simulink model "blockdemo_preaddermodes"  (Simulink 7.6)
settings: Solver=ode45  StartTime=0.0  StopTime=10.0  RelTol=1e-3
InitFcn:
  | %% DSPBuilder Start
  | alt_dspbuilder_update_model(bdroot)
  | %% DSPBuilder End
libraries: allblocks_alteradspbuilder2 x19
settings Model: Creator=akarapet  LastModifiedBy=akarapet

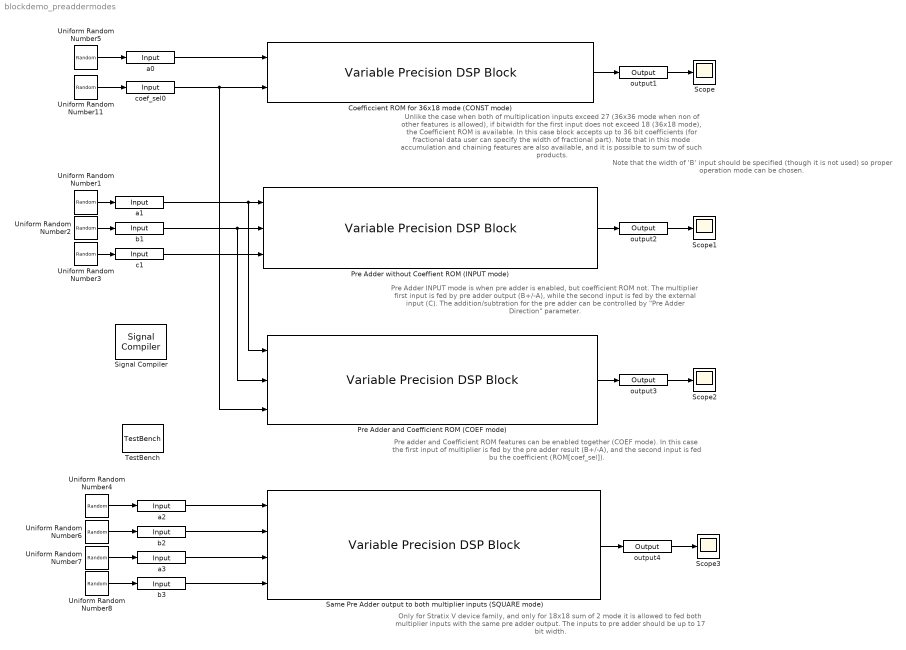
== system blockdemo_preaddermodes ==
  note: Unlike the case when both of multiplication inputs exceed 27 (36x36 mode when non of other features is allowed),
      | if bitwidth for the first input does not exceed 18 (36x18 mode), the Coefficient ROM is available.
      | In this case block accepts up to 36 bit coefficients (for fractional data user can specify the width of fractional part).
      | Note that in this mode accumulation and chaining features are also available, and it is possible to sum tw of such products.
  note: Note that the width of 'B' input should be specified (though it is not used) so proper operation mode can be chosen.
  note: Pre Adder INPUT mode is when pre adder is enabled, but coefficient ROM not. The multiplier first input is fed by
      | pre adder output (B+/-A), while the second input is fed by the external input (C).
      | The addition/subtration for the pre adder can be controlled by "Pre Adder Direction" parameter.
  note: Pre adder and Coefficient ROM features can be enabled together (COEF mode). In this case the first input
      | of multiplier is fed by the pre adder result (B+/-A), and the second input is fed bu the coefficient (ROM[coef_sel]).
  note: Only for Stratix V device family, and only for 18x18 sum of 2 mode it is allowed to fed
      | both multiplier inputs with the same pre adder output.
      | The inputs to pre adder should be up to 17 bit width.
  Coefficcient ROM for 36x18 mode (CONST mode) : allblocks_alteradspbuilder2/Variable Precision DSP Block  complex_model_delayed=0  model_delayed=0  device_family=Stratix V  used_mode_stratix=Other Modes  used_mode_arria=Other Modes  in_25x18_complex_mode=0  in_18x18plus36_mode=0  in_other_modes=1  number_of_mults=1  clock_ena_inputs=off  async_clear_inputs=off  bus_type=Signed Integer  bwl_A=18  bwr_A=0  width_A=18  chain_width=64  reg_inputs_A=off  A_inputs_reg_ena=ENABLE 0  bwl_B=36  bwr_B=0  width_B=36  reg_inputs_B=off  B_inputs_reg_ena=ENABLE 0  bwl_joint_A_B=8  bwr_joint_A_B=0  reg_joint_A_B_input=on  A_B_input_reg_ena=ENABLE 0  bwl_A_complex=8  bwr_A_complex=8  reg_complex_A=on  A_complex_inputs_reg_ena=ENABLE 0  bwl_B_complex=8  bwr_B_complex=8  reg_complex_B=on  B_complex_inputs_reg_ena=ENABLE 0  A_inputs_exist=1  B_inputs_exist=0  C_inputs_exist=0  coef_sel_inputs_exist=1  all_inputs_registered=0  no_input_registered=1  all_inputs_share_same_clocks=1  full_resolution=off  bwl_out=54  bwr_out=0  reg_output=off  output_reg_ena=ENABLE 0  systolic_regs_available=0  enable_systolic_regs=off  systolic_regs_used=0  basic_struct_ok_for_input_scan=0  input_scan_available=0  enable_input_scan=off  input_scan_used=0  input_scan_delay_regs_available=0  enable_input_scan_delay_regs=off  input_scan_delay_regs_used=0  basic_struct_ok_for_coef_rom=1  coef_rom_available=1  enable_coef_rom=on  coef_rom_used=1  basic_struct_ok_for_preadder=0  preadder_available=0  enable_preadder=off  preadder_used=0  preadder_direction=ADD  square_mode_available=0  enable_square_mode=off  square_mode_used=0  upper_limit_9bit=9  upper_limit_18bit=18  upper_limit_27bit=27  in_18x18_modes=0  in_27x27_modes=0  in_36x18_modes=1  in_36x36_mode=0  mult1_adder_available=0  mult1_direction=ADD  mult3_adder_available=0  mult3_direction=ADD  chainout_adder_available=1  use_chainout_input=off  chainout_input_used=0  use_chainout_output=off  chainout_output_used=0  accum_available=1  enable_accum=off  accum_used=0  double_accum_available=0  enable_double_accum=off  double_accum_used=0  negate_available=1  mult_add_operation=ADD  rounding_constant_available=1  use_rounding_constant=off  rounding_constant_used=0  constant_value=1  bwl_C=8  bwr_C=0  bwl_coef=36  bwr_coef=0  mult0_coeffs=[2147483648, -2147483648, -211, 0, 7, 44, -2147483630, 333]  mult1_coeffs=[0, 0, 0, 0, 0, 0, 0, 0]  mult2_coeffs=[0, 0, 0, 0, 0, 0, 0, 0]  mult3_coeffs=[0, 0, 0, 0, 0, 0, 0, 0]  reg_mult1_op_control=off  reg_mult3_op_control=off  reg_accum_control=off  reg_negate_control=off  control_regs_ena=ENABLE 0
  Pre Adder and Coefficient ROM (COEF mode) : allblocks_alteradspbuilder2/Variable Precision DSP Block  complex_model_delayed=0  model_delayed=0  device_family=Stratix V  used_mode_stratix=Other Modes  used_mode_arria=Other Modes  in_25x18_complex_mode=0  in_18x18plus36_mode=0  in_other_modes=1  number_of_mults=1  clock_ena_inputs=off  async_clear_inputs=off  bus_type=Signed Integer  bwl_A=20  bwr_A=0  width_A=20  chain_width=64  reg_inputs_A=on  A_inputs_reg_ena=ENABLE 0  bwl_B=20  bwr_B=0  width_B=20  reg_inputs_B=on  B_inputs_reg_ena=ENABLE 0  bwl_joint_A_B=8  bwr_joint_A_B=0  reg_joint_A_B_input=on  A_B_input_reg_ena=ENABLE 0  bwl_A_complex=8  bwr_A_complex=8  reg_complex_A=on  A_complex_inputs_reg_ena=ENABLE 0  bwl_B_complex=8  bwr_B_complex=8  reg_complex_B=on  B_complex_inputs_reg_ena=ENABLE 0  A_inputs_exist=1  B_inputs_exist=1  C_inputs_exist=0  coef_sel_inputs_exist=1  all_inputs_registered=1  no_input_registered=0  all_inputs_share_same_clocks=1  full_resolution=off  bwl_out=41  bwr_out=0  reg_output=off  output_reg_ena=ENABLE 0  systolic_regs_available=0  enable_systolic_regs=off  systolic_regs_used=0  basic_struct_ok_for_input_scan=1  input_scan_available=0  enable_input_scan=off  input_scan_used=0  input_scan_delay_regs_available=0  enable_input_scan_delay_regs=off  input_scan_delay_regs_used=0  basic_struct_ok_for_coef_rom=1  coef_rom_available=1  enable_coef_rom=on  coef_rom_used=1  basic_struct_ok_for_preadder=1  preadder_available=1  enable_preadder=on  preadder_used=1  preadder_direction=ADD  square_mode_available=0  enable_square_mode=off  square_mode_used=0  upper_limit_9bit=9  upper_limit_18bit=17  upper_limit_27bit=27  in_18x18_modes=0  in_27x27_modes=1  in_36x18_modes=0  in_36x36_mode=0  mult1_adder_available=0  mult1_direction=ADD  mult3_adder_available=0  mult3_direction=ADD  chainout_adder_available=1  use_chainout_input=off  chainout_input_used=0  use_chainout_output=off  chainout_output_used=0  accum_available=1  enable_accum=off  accum_used=0  double_accum_available=0  enable_double_accum=off  double_accum_used=0  negate_available=1  mult_add_operation=ADD  rounding_constant_available=1  use_rounding_constant=off  rounding_constant_used=0  constant_value=1  bwl_C=20  bwr_C=0  bwl_coef=27  bwr_coef=0  mult0_coeffs=[200, -38, 21, -76, 7, 44, -1, 0]  mult1_coeffs=[0, 0, 0, 0, 0, 0, 0, 0]  mult2_coeffs=[0, 0, 0, 0, 0, 0, 0, 0]  mult3_coeffs=[0, 0, 0, 0, 0, 0, 0, 0]  reg_mult1_op_control=off  reg_mult3_op_control=off  reg_accum_control=off  reg_negate_control=off  control_regs_ena=ENABLE 0
  Pre Adder without Coeffient ROM (INPUT mode) : allblocks_alteradspbuilder2/Variable Precision DSP Block  complex_model_delayed=0  model_delayed=0  device_family=Stratix V  used_mode_stratix=Other Modes  used_mode_arria=Other Modes  in_25x18_complex_mode=0  in_18x18plus36_mode=0  in_other_modes=1  number_of_mults=1  clock_ena_inputs=off  async_clear_inputs=off  bus_type=Signed Integer  bwl_A=20  bwr_A=0  width_A=20  chain_width=64  reg_inputs_A=on  A_inputs_reg_ena=ENABLE 0  bwl_B=20  bwr_B=0  width_B=20  reg_inputs_B=on  B_inputs_reg_ena=ENABLE 0  bwl_joint_A_B=8  bwr_joint_A_B=0  reg_joint_A_B_input=on  A_B_input_reg_ena=ENABLE 0  bwl_A_complex=8  bwr_A_complex=8  reg_complex_A=on  A_complex_inputs_reg_ena=ENABLE 0  bwl_B_complex=8  bwr_B_complex=8  reg_complex_B=on  B_complex_inputs_reg_ena=ENABLE 0  A_inputs_exist=1  B_inputs_exist=1  C_inputs_exist=1  coef_sel_inputs_exist=0  all_inputs_registered=1  no_input_registered=0  all_inputs_share_same_clocks=1  full_resolution=off  bwl_out=41  bwr_out=0  reg_output=on  output_reg_ena=ENABLE 0  systolic_regs_available=0  enable_systolic_regs=off  systolic_regs_used=0  basic_struct_ok_for_input_scan=1  input_scan_available=0  enable_input_scan=off  input_scan_used=0  input_scan_delay_regs_available=0  enable_input_scan_delay_regs=off  input_scan_delay_regs_used=0  basic_struct_ok_for_coef_rom=1  coef_rom_available=1  enable_coef_rom=off  coef_rom_used=0  basic_struct_ok_for_preadder=1  preadder_available=1  enable_preadder=on  preadder_used=1  preadder_direction=ADD  square_mode_available=0  enable_square_mode=off  square_mode_used=0  upper_limit_9bit=9  upper_limit_18bit=17  upper_limit_27bit=27  in_18x18_modes=0  in_27x27_modes=1  in_36x18_modes=0  in_36x36_mode=0  mult1_adder_available=0  mult1_direction=ADD  mult3_adder_available=0  mult3_direction=ADD  chainout_adder_available=1  use_chainout_input=off  chainout_input_used=0  use_chainout_output=off  chainout_output_used=0  accum_available=1  enable_accum=off  accum_used=0  double_accum_available=0  enable_double_accum=off  double_accum_used=0  negate_available=1  mult_add_operation=ADD  rounding_constant_available=1  use_rounding_constant=off  rounding_constant_used=0  constant_value=1  bwl_C=20  bwr_C=0  bwl_coef=27  bwr_coef=0  mult0_coeffs=[0, 0, 0, 0, 0, 0, 0, 0]  mult1_coeffs=[0, 0, 0, 0, 0, 0, 0, 0]  mult2_coeffs=[0, 0, 0, 0, 0, 0, 0, 0]  mult3_coeffs=[0, 0, 0, 0, 0, 0, 0, 0]  reg_mult1_op_control=off  reg_mult3_op_control=off  reg_accum_control=off  reg_negate_control=off  control_regs_ena=ENABLE 0
  Same Pre Adder output to both multiplier inputs (SQUARE mode) : allblocks_alteradspbuilder2/Variable Precision DSP Block  complex_model_delayed=0  model_delayed=0  device_family=Stratix V  used_mode_stratix=Other Modes  used_mode_arria=Other Modes  in_25x18_complex_mode=0  in_18x18plus36_mode=0  in_other_modes=1  number_of_mults=2  clock_ena_inputs=off  async_clear_inputs=off  bus_type=Signed Integer  bwl_A=17  bwr_A=0  width_A=17  chain_width=64  reg_inputs_A=off  A_inputs_reg_ena=ENABLE 0  bwl_B=17  bwr_B=0  width_B=17  reg_inputs_B=off  B_inputs_reg_ena=ENABLE 0  bwl_joint_A_B=8  bwr_joint_A_B=0  reg_joint_A_B_input=on  A_B_input_reg_ena=ENABLE 0  bwl_A_complex=8  bwr_A_complex=8  reg_complex_A=on  A_complex_inputs_reg_ena=ENABLE 0  bwl_B_complex=8  bwr_B_complex=8  reg_complex_B=on  B_complex_inputs_reg_ena=ENABLE 0  A_inputs_exist=1  B_inputs_exist=1  C_inputs_exist=0  coef_sel_inputs_exist=0  all_inputs_registered=0  no_input_registered=1  all_inputs_share_same_clocks=1  full_resolution=off  bwl_out=35  bwr_out=0  reg_output=on  output_reg_ena=ENABLE 0  systolic_regs_available=1  enable_systolic_regs=off  systolic_regs_used=0  basic_struct_ok_for_input_scan=1  input_scan_available=0  enable_input_scan=off  input_scan_used=0  input_scan_delay_regs_available=0  enable_input_scan_delay_regs=off  input_scan_delay_regs_used=0  basic_struct_ok_for_coef_rom=1  coef_rom_available=1  enable_coef_rom=off  coef_rom_used=0  basic_struct_ok_for_preadder=1  preadder_available=1  enable_preadder=on  preadder_used=1  preadder_direction=SUB  square_mode_available=1  enable_square_mode=on  square_mode_used=1  upper_limit_9bit=9  upper_limit_18bit=17  upper_limit_27bit=27  in_18x18_modes=1  in_27x27_modes=0  in_36x18_modes=0  in_36x36_mode=0  mult1_adder_available=1  mult1_direction=ADD  mult3_adder_available=0  mult3_direction=ADD  chainout_adder_available=1  use_chainout_input=off  chainout_input_used=0  use_chainout_output=off  chainout_output_used=0  accum_available=1  enable_accum=off  accum_used=0  double_accum_available=0  enable_double_accum=off  double_accum_used=0  negate_available=1  mult_add_operation=ADD  rounding_constant_available=1  use_rounding_constant=off  rounding_constant_used=0  constant_value=1  bwl_C=20  bwr_C=0  bwl_coef=18  bwr_coef=0  mult0_coeffs=[200, -38, 21, -76, 7, 44, -1, 0]  mult1_coeffs=[0, 0, 0, 0, 0, 0, 0, 0]  mult2_coeffs=[0, 0, 0, 0, 0, 0, 0, 0]  mult3_coeffs=[0, 0, 0, 0, 0, 0, 0, 0]  reg_mult1_op_control=off  reg_mult3_op_control=off  reg_accum_control=off  reg_negate_control=off  control_regs_ena=ENABLE 0
  Scope{,1..3} (4 alike) : Scope
      Scope2 settings: SaveName=ScopeData2
      Scope3 settings: SaveName=ScopeData3
  Signal Compiler : allblocks_alteradspbuilder2/Signal Compiler  DeviceFamily=Stratix V  DeviceName=AUTO  EnableSignalTap=off  SignalTapDepth=128  UseBoardBlock=off  StpUseDefaultClock=on  StpClock=Clock  ExportDir=<binary blob, 153 chars, not shown>
  TestBench : allblocks_alteradspbuilder2/TestBench  enable=on  advancedMode=off  modelSimGui=off  maxDisplayErrors=10  mismatchErrorLevel=Error  simdatafile=/data/akarapet/qshell_linux64_regtests/p4/dsp_builder/dsp_builder2/Documentation/DesignExamples/Tutorials/UnitBlocks/Arithmetic/VariablePrecisionDSPBlock/tb_blockdemo_preaddermodes/blockdemo_preaddermodes.simdata.tcl
  Uniform Random Number{1,4..8} (6 alike) : UniformRandomNumber  Minimum=-2147483642  Maximum=2147483642  Seed=1591  SampleTime=1
  Uniform Random Number11 : UniformRandomNumber  Minimum=0  Maximum=7  Seed=1591  SampleTime=1
  Uniform Random Number2 : UniformRandomNumber  Minimum=-2147483642  Maximum=2147483642  Seed=3333  SampleTime=1
  Uniform Random Number3 : UniformRandomNumber  Minimum=-2147483642  Maximum=2147483642  Seed=3323  SampleTime=1
  a0 : allblocks_alteradspbuilder2/Input  iofile=/data/akarapet/qshell_linux64_regtests/p4/dsp_builder/dsp_builder2/Documentation/DesignExamples/Tutorials/UnitBlocks/Arithmetic/VariablePrecisionDSPBlock/tb_blockdemo_preaddermodes/blockdemo%5Fpreaddermodes_a0.salt  BusType=Signed Integer  bwl=18  bwr=0  SpecifyClock=off  clock=default_clock  PORTTYPE=Input  externalType=Inferred  allowFloatingPointOverride=on  logOutputs=off
  a1 : allblocks_alteradspbuilder2/Input  iofile=/data/akarapet/qshell_linux64_regtests/p4/dsp_builder/dsp_builder2/Documentation/DesignExamples/Tutorials/UnitBlocks/Arithmetic/VariablePrecisionDSPBlock/tb_blockdemo_preaddermodes/blockdemo%5Fpreaddermodes_a1.salt  BusType=Signed Integer  bwl=20  bwr=0  SpecifyClock=off  clock=default_clock  PORTTYPE=Input  externalType=Inferred  allowFloatingPointOverride=on  logOutputs=off
  a2 : allblocks_alteradspbuilder2/Input  iofile=/data/akarapet/qshell_linux64_regtests/p4/dsp_builder/dsp_builder2/Documentation/DesignExamples/Tutorials/UnitBlocks/Arithmetic/VariablePrecisionDSPBlock/tb_blockdemo_preaddermodes/blockdemo%5Fpreaddermodes_a2.salt  BusType=Signed Integer  bwl=17  bwr=0  SpecifyClock=off  clock=default_clock  PORTTYPE=Input  externalType=Inferred  allowFloatingPointOverride=on  logOutputs=off
  a3 : allblocks_alteradspbuilder2/Input  iofile=/data/akarapet/qshell_linux64_regtests/p4/dsp_builder/dsp_builder2/Documentation/DesignExamples/Tutorials/UnitBlocks/Arithmetic/VariablePrecisionDSPBlock/tb_blockdemo_preaddermodes/blockdemo%5Fpreaddermodes_a3.salt  BusType=Signed Integer  bwl=17  bwr=0  SpecifyClock=off  clock=default_clock  PORTTYPE=Input  externalType=Inferred  allowFloatingPointOverride=on  logOutputs=off
  b1 : allblocks_alteradspbuilder2/Input  iofile=/data/akarapet/qshell_linux64_regtests/p4/dsp_builder/dsp_builder2/Documentation/DesignExamples/Tutorials/UnitBlocks/Arithmetic/VariablePrecisionDSPBlock/tb_blockdemo_preaddermodes/blockdemo%5Fpreaddermodes_b1.salt  BusType=Signed Integer  bwl=20  bwr=0  SpecifyClock=off  clock=default_clock  PORTTYPE=Input  externalType=Inferred  allowFloatingPointOverride=on  logOutputs=off
  b2 : allblocks_alteradspbuilder2/Input  iofile=/data/akarapet/qshell_linux64_regtests/p4/dsp_builder/dsp_builder2/Documentation/DesignExamples/Tutorials/UnitBlocks/Arithmetic/VariablePrecisionDSPBlock/tb_blockdemo_preaddermodes/blockdemo%5Fpreaddermodes_b2.salt  BusType=Signed Integer  bwl=17  bwr=0  SpecifyClock=off  clock=default_clock  PORTTYPE=Input  externalType=Inferred  allowFloatingPointOverride=on  logOutputs=off
  b3 : allblocks_alteradspbuilder2/Input  iofile=/data/akarapet/qshell_linux64_regtests/p4/dsp_builder/dsp_builder2/Documentation/DesignExamples/Tutorials/UnitBlocks/Arithmetic/VariablePrecisionDSPBlock/tb_blockdemo_preaddermodes/blockdemo%5Fpreaddermodes_b3.salt  BusType=Signed Integer  bwl=17  bwr=0  SpecifyClock=off  clock=default_clock  PORTTYPE=Input  externalType=Inferred  allowFloatingPointOverride=on  logOutputs=off
  c1 : allblocks_alteradspbuilder2/Input  iofile=/data/akarapet/qshell_linux64_regtests/p4/dsp_builder/dsp_builder2/Documentation/DesignExamples/Tutorials/UnitBlocks/Arithmetic/VariablePrecisionDSPBlock/tb_blockdemo_preaddermodes/blockdemo%5Fpreaddermodes_c1.salt  BusType=Signed Integer  bwl=20  bwr=0  SpecifyClock=off  clock=default_clock  PORTTYPE=Input  externalType=Inferred  allowFloatingPointOverride=on  logOutputs=off
  coef_sel0 : allblocks_alteradspbuilder2/Input  iofile=/data/akarapet/qshell_linux64_regtests/p4/dsp_builder/dsp_builder2/Documentation/DesignExamples/Tutorials/UnitBlocks/Arithmetic/VariablePrecisionDSPBlock/tb_blockdemo_preaddermodes/blockdemo%5Fpreaddermodes_coef%5Fsel0.salt  BusType=Unsigned Integer  bwl=3  bwr=0  SpecifyClock=off  clock=default_clock  PORTTYPE=Input  externalType=Inferred  allowFloatingPointOverride=on  logOutputs=off
  output1 : allblocks_alteradspbuilder2/Output  iofile=/data/akarapet/qshell_linux64_regtests/p4/dsp_builder/dsp_builder2/Documentation/DesignExamples/Tutorials/UnitBlocks/Arithmetic/VariablePrecisionDSPBlock/tb_blockdemo_preaddermodes/blockdemo%5Fpreaddermodes_output1.capture  BusType=Signed Integer  bwl=54  bwr=0  externalType=Inferred  PORTTYPE=Output  allowFloatingPointOverride=on  logOutputs=off
  output2 : allblocks_alteradspbuilder2/Output  iofile=/data/akarapet/qshell_linux64_regtests/p4/dsp_builder/dsp_builder2/Documentation/DesignExamples/Tutorials/UnitBlocks/Arithmetic/VariablePrecisionDSPBlock/tb_blockdemo_preaddermodes/blockdemo%5Fpreaddermodes_output2.capture  BusType=Signed Integer  bwl=41  bwr=0  externalType=Inferred  PORTTYPE=Output  allowFloatingPointOverride=on  logOutputs=off
  output3 : allblocks_alteradspbuilder2/Output  iofile=/data/akarapet/qshell_linux64_regtests/p4/dsp_builder/dsp_builder2/Documentation/DesignExamples/Tutorials/UnitBlocks/Arithmetic/VariablePrecisionDSPBlock/tb_blockdemo_preaddermodes/blockdemo%5Fpreaddermodes_output3.capture  BusType=Signed Integer  bwl=41  bwr=0  externalType=Inferred  PORTTYPE=Output  allowFloatingPointOverride=on  logOutputs=off
  output4 : allblocks_alteradspbuilder2/Output  iofile=/data/akarapet/qshell_linux64_regtests/p4/dsp_builder/dsp_builder2/Documentation/DesignExamples/Tutorials/UnitBlocks/Arithmetic/VariablePrecisionDSPBlock/tb_blockdemo_preaddermodes/blockdemo%5Fpreaddermodes_output4.capture  BusType=Signed Integer  bwl=35  bwr=0  externalType=Inferred  PORTTYPE=Output  allowFloatingPointOverride=on  logOutputs=off
  wires:
  a0/1 -> Coefficcient ROM for 36x18 mode (CONST mode)/1
  Uniform Random Number11/1 -> coef_sel0/1
  Uniform Random Number5/1 -> a0/1
  coef_sel0/1 -> Coefficcient ROM for 36x18 mode (CONST mode)/2, Pre Adder and Coefficient ROM (COEF mode)/3
  Coefficcient ROM for 36x18 mode (CONST mode)/1 -> output1/1
  output1/1 -> Scope/1
  a1/1 -> Pre Adder without Coeffient ROM (INPUT mode)/1, Pre Adder and Coefficient ROM (COEF mode)/1
  b1/1 -> Pre Adder without Coeffient ROM (INPUT mode)/2, Pre Adder and Coefficient ROM (COEF mode)/2
  c1/1 -> Pre Adder without Coeffient ROM (INPUT mode)/3
  Uniform Random Number1/1 -> a1/1
  Uniform Random Number2/1 -> b1/1
  Uniform Random Number3/1 -> c1/1
  Pre Adder without Coeffient ROM (INPUT mode)/1 -> output2/1
  output2/1 -> Scope1/1
  Pre Adder and Coefficient ROM (COEF mode)/1 -> output3/1
  output3/1 -> Scope2/1
  Same Pre Adder output to both multiplier inputs (SQUARE mode)/1 -> output4/1
  output4/1 -> Scope3/1
  Uniform Random Number4/1 -> a2/1
  Uniform Random Number6/1 -> b2/1
  Uniform Random Number7/1 -> a3/1
  Uniform Random Number8/1 -> b3/1
  a2/1 -> Same Pre Adder output to both multiplier inputs (SQUARE mode)/1
  b2/1 -> Same Pre Adder output to both multiplier inputs (SQUARE mode)/2
  a3/1 -> Same Pre Adder output to both multiplier inputs (SQUARE mode)/3
  b3/1 -> Same Pre Adder output to both multiplier inputs (SQUARE mode)/4
